simulink model "moj_statek2"  (R2016a)
settings: Solver=VariableStepAuto  StartTime=0.0  StopTime=3000.0  RelTol=1e-3
settings Model: Creator=za32917  LastModifiedBy=za32917

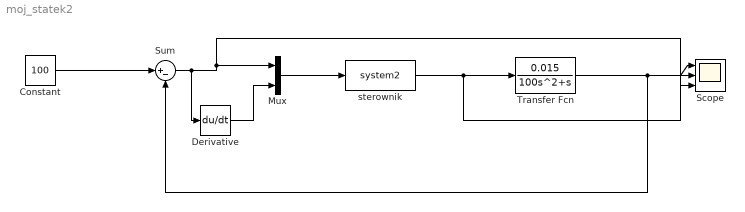
== system moj_statek2 ==
  Constant : Constant  Value=100
  Derivative : Derivative
  Mux : Mux  Inputs=2
  Scope : Scope  NumInputPorts=3
  Sum : Sum  Inputs=|+-
  Transfer Fcn : TransferFcn  Numerator=0.015  Denominator=[100,1,0]
  "sterownik " : MATLABFcn  MATLABFcn=system2
  wires:
  "sterownik "/1 -> Scope/2, Transfer Fcn/1
  Transfer Fcn/1 -> Sum/2, Scope/1
  Constant/1 -> Sum/1
  Sum/1 -> Derivative/1, Mux/1, Scope/3
  Mux/1 -> "sterownik "/1
  Derivative/1 -> Mux/2
